simulink model "Group_28_Milestone1"  (R2020a)
settings: Solver=VariableStepAuto  StartTime=0.0  StopTime=3  RelTol=1e-3
libraries: simulink x4
settings Model: Creator=matthewterblanche  LastModifiedBy=matthewterblanche

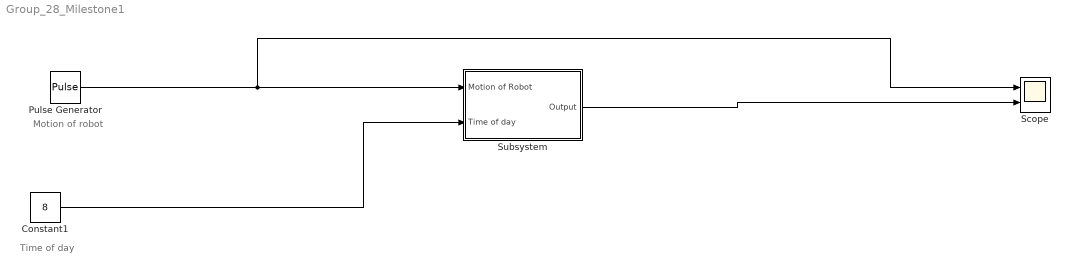
== system Group_28_Milestone1 ==
  note: Motion of robot
  note: Time of day
  Constant1 : Constant  Value=8
  Pulse Generator : DiscretePulseGenerator  PulseType=Time based  Period=0.4  PulseWidth=50  PhaseDelay=0.2
  Scope : Scope  NumInputPorts=2
  Subsystem : Subsystem
  wires:
  Pulse Generator/1 -> Scope/1, Subsystem/1(Motion of Robot)
  Constant1/1 -> Subsystem/2(Time of day)
  Subsystem/1(Output) -> Scope/2

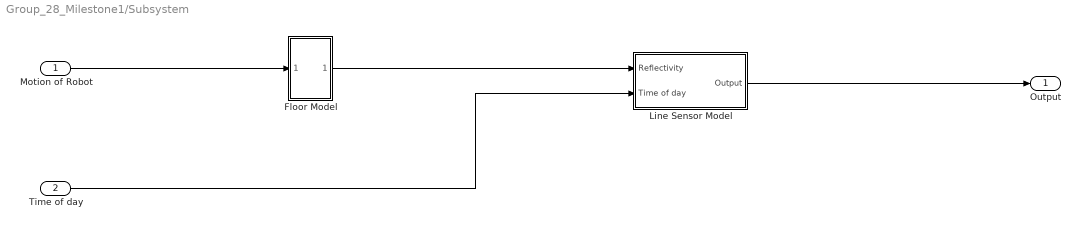
== system Group_28_Milestone1/Subsystem ==
  Motion of Robot : Inport
  Time of day : Inport  Port=2
  Floor Model : Subsystem
  Line Sensor Model : Subsystem
  Output : Outport
  wires:
  Line Sensor Model/1(Output) -> Output/1
  Time of day/1 -> Line Sensor Model/2(Time of day)
  Motion of Robot/1 -> Floor Model/1(In1)
  Floor Model/1(Out1) -> Line Sensor Model/1(Reflectivity)

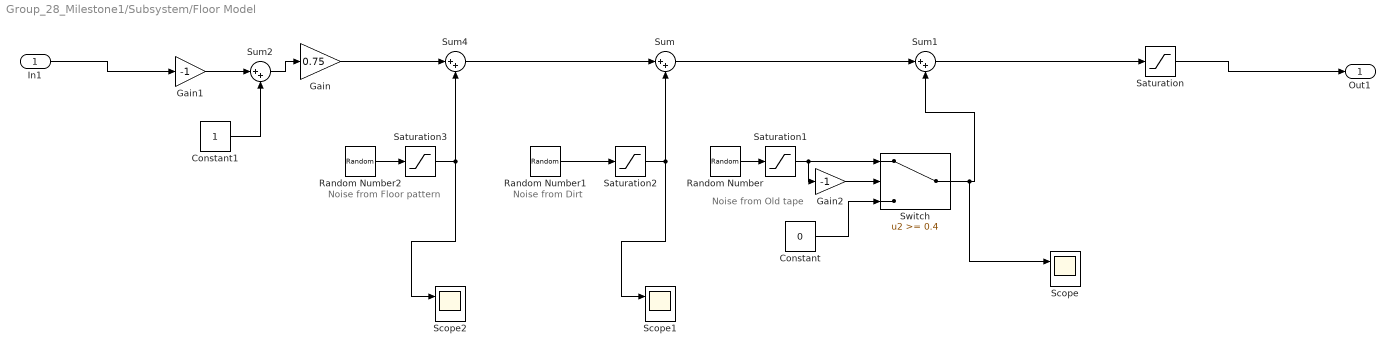
== system Group_28_Milestone1/Subsystem/Floor Model ==
  note: Noise from
      | Old tape
  note: Noise from Dirt
  note: Noise from Floor pattern
  In1 : Inport
  Constant : Constant  Value=0
  Constant1 : Constant
  Gain : Gain  Gain=0.75
  Gain1 : Gain  Gain=-1
  Gain2 : Gain  Gain=-1
  Random Number : RandomNumber  Variance=0.06  Seed=123  SampleTime=0.2
  Random Number1 : RandomNumber  Variance=0.01  Seed=124  SampleTime=0.01
  Random Number2 : RandomNumber  Variance=0.1  Seed=100  SampleTime=0.01
  Saturation : Saturate  UpperLimit=1  LowerLimit=0
  Saturation1 : Saturate  UpperLimit=0  LowerLimit=-0.6
  Saturation2 : Saturate  UpperLimit=0.1  LowerLimit=-0.1
  Saturation3 : Saturate  UpperLimit=0.05  LowerLimit=-0.05
  Scope : Scope  NumInputPorts=2
  Scope1 : Scope  NumInputPorts=2
  Scope2 : Scope  NumInputPorts=2
  Sum{,1..2,4} (4 alike) : Sum  Inputs=|++
  Switch : Switch  Threshold=0.4
  Out1 : Outport
  wires:
  Sum2/1 -> Gain/1
  Gain1/1 -> Sum2/1
  Gain/1 -> Sum4/1
  Constant1/1 -> Sum2/2
  Saturation/1 -> Out1/1
  In1/1 -> Gain1/1
  Sum/1 -> Sum1/1
  Random Number1/1 -> Saturation2/1
  Random Number/1 -> Saturation1/1
  Constant/1 -> Switch/3
  Saturation1/1 -> Switch/1, Gain2/1
  Gain2/1 -> Switch/2
  Switch/1 -> Scope/1, Sum1/2
  Saturation2/1 -> Scope1/1, Sum/2
  Random Number2/1 -> Saturation3/1
  Saturation3/1 -> Scope2/1, Sum4/2
  Sum4/1 -> Sum/1
  Sum1/1 -> Saturation/1

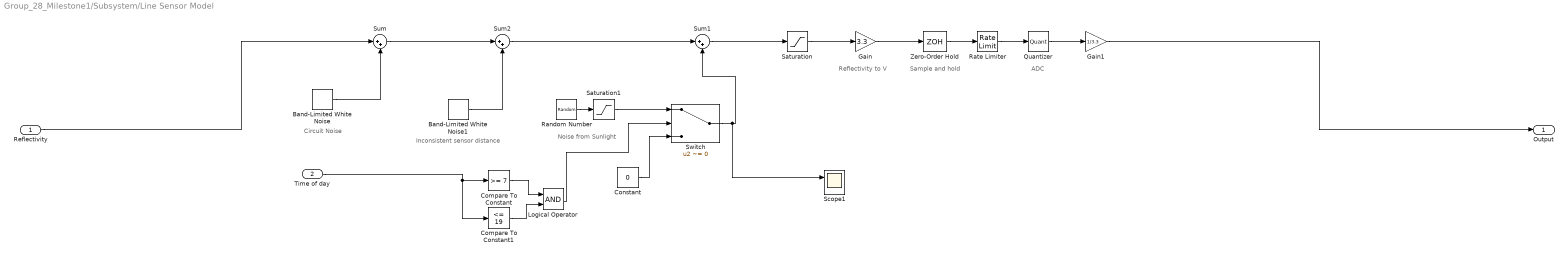
== system Group_28_Milestone1/Subsystem/Line Sensor Model ==
  note: Inconsistent sensor distance
  note: Noise from
      | Sunlight
  note: Circuit Noise
  note: Reflectivity to V
  note: Sample and hold
  note: ADC
  Reflectivity : Inport
  Time of day : Inport  Port=2
  Band-Limited White Noise : simulink/Sources/Band-Limited White Noise  Cov=1/1000*(0.01)^2  Ts=1/1000  seed=[23341]
  Band-Limited White Noise1 : simulink/Sources/Band-Limited White Noise  Cov=1/1000*(0.02)^2  Ts=1/1000  seed=[23341]
  Compare To Constant : simulink/Logic and Bit Operations/Compare To Constant  relop=>=  const=7  OutDataTypeStr=boolean
  Compare To Constant1 : simulink/Logic and Bit Operations/Compare To Constant  relop=<=  const=19  OutDataTypeStr=boolean
  Constant : Constant  Value=0
  Gain : Gain  Gain=3.3
  Gain1 : Gain  Gain=1/3.3
  Logical Operator : Logic  AllPortsSameDT=off  OutDataTypeStr=boolean
  Quantizer : Quantizer  QuantizationInterval=3.3/((2^12)-1)
  Random Number : RandomNumber  Variance=0.06  Seed=140  SampleTime=0.01
  Rate Limiter : RateLimiter  RisingSlewLimit=3.3/(10*10^(-6))  FallingSlewLimit=-3.3/(50*10^(-6))  SampleTimeMode=inherited
  Saturation : Saturate  UpperLimit=3.3  LowerLimit=0
  Saturation1 : Saturate  UpperLimit=0.02  LowerLimit=0
  Scope1 : Scope  NumInputPorts=2
  Sum : Sum  Inputs=|++
  Sum1 : Sum  Inputs=|++
  Sum2 : Sum  Inputs=|++
  Switch : Switch  Criteria=u2 ~= 0  Threshold=0.4
  Zero-Order Hold : ZeroOrderHold  SampleTime=1/100
  Output : Outport
  wires:
  Reflectivity/1 -> Sum/1
  Random Number/1 -> Saturation1/1
  Quantizer/1 -> Gain1/1
  Saturation/1 -> Gain/1
  Constant/1 -> Switch/3
  Sum/1 -> Sum2/1
  Gain/1 -> Zero-Order Hold/1
  Compare To Constant1/1 -> Logical Operator/2
  Band-Limited White Noise/1 -> Sum/2
  Compare To Constant/1 -> Logical Operator/1
  Rate Limiter/1 -> Quantizer/1
  Time of day/1 -> Compare To Constant1/1, Compare To Constant/1
  Gain1/1 -> Output/1
  Sum1/1 -> Saturation/1
  Saturation1/1 -> Switch/1
  Zero-Order Hold/1 -> Rate Limiter/1
  Switch/1 -> Scope1/1, Sum1/2
  Logical Operator/1 -> Switch/2
  Sum2/1 -> Sum1/1
  Band-Limited White Noise1/1 -> Sum2/2
